simulink model "xpcserialbinarytest_orig"  (Simulink 7.1)
settings: Solver=FixedStepDiscrete  StartTime=0.0  StopTime=inf  RelTol=1e-3
InitFcn:
  | trun = .01;
libraries: xpclib x5, xpcutilitieslib x2, simulink x1
Description:
  | Serial Blocks Loopback Test Using Binary Encoding/Decoding
  | 
  | This model demonstrates the BINARY FIFO read block in a form that can be simulated without using any specific serial hardware.  The input to the FIFO write block is the concatenation of several pieces comprising two separate 'messages'.  The first message is the byte stream: [170, 1, N] and the second is [170 2 44 M] where N is an incrementing number and M is a decrementing number.  The initial '8' in the first constant is the number of elements that follow.  The '5' is an extraneous value that shows how the FIFO binary read will ignore extra information.
  | 
  | To run this test with real serial port hardware, replace the FIFO write block with the send/receive block with FIFO OUT that corresponds to your hardware from the xpclib rs232 section. Then feed the output signal back to the input with a wire to perform a loopback test.
settings Model: Creator=gweast  LastModifiedBy=Administrator  ExtModeArmWhenConnect=off  BufferReuse=off
settings DataIOCC: SaveOutput=off  SignalLogging=off  SaveTime=off
settings OptimizationCC: BlockReduction=off  OptimizeBlockIOStorage=off  BufferReuse=off  ExpressionFolding=off  FoldNonRolledExpr=off  LocalBlockOutputs=off
settings DebuggingCC: SaveWithParameterizedLinksMsg=none  SignalResolutionControl=TryResolveAllWithWarning  MultiTaskDSMMsg=warning  MultiTaskCondExecSysMsg=none  StrictBusMsg=None
settings HardwareCC: ProdIntDivRoundTo=Zero  ProdEndianess=LittleEndian  ProdHWDeviceType=Generic->32-bit x86 compatible
settings RTWCC: SystemTargetFile=xpctarget.tlc  TemplateMakefile=xpc_default_tmf  Description=xPC Target  ProcessScript=xpctarget_make_rtw_hook  IncludeERTFirstTime=on
settings xpcTargetCC: TargetFcnLib=ansi_tfl_tmw.mat  TargetFunctionLibrary=ANSI_C  CompOptLevelCompliant=off  PortableWordSizes=off  xPCisDownloadable=off

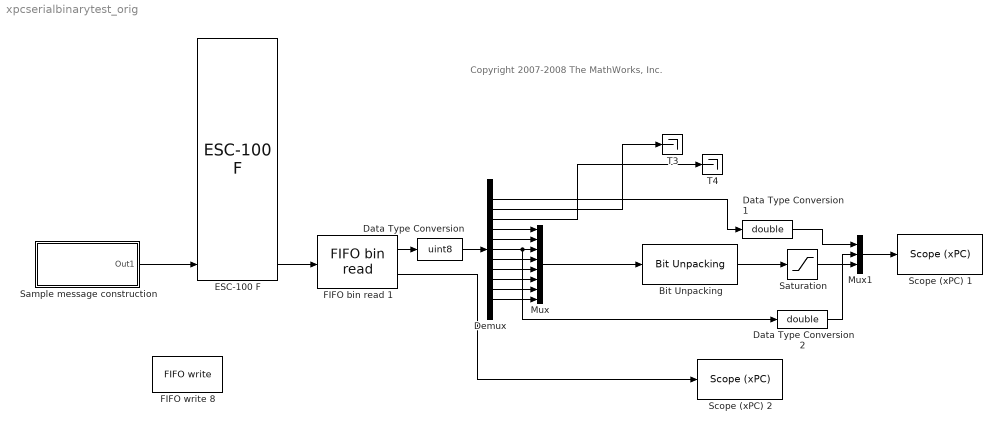
== system xpcserialbinarytest_orig ==
  note: Copyright 2007-2008 The MathWorks, Inc.
  "Bit Unpacking " : xpcutilitieslib/Bit Unpacking   SignExtend=off  MaskBitPatterns={[0:63]}  MaskPackDataType=uint8  MaskPackDataSize=[8]  MaskUnpackDataTypes={'double'}  MaskUnpackDataSizes={[1]}
  Data Type Conversion : DataTypeConversion  OutDataTypeMode=uint8  OutDataType=sfix(16)  OutScaling=2^0  OutDataTypeStr=uint8
  Data Type Conversion1 : DataTypeConversion  OutDataTypeMode=double  OutDataType=sfix(16)  OutScaling=2^0  OutDataTypeStr=double
  Data Type Conversion2 : DataTypeConversion  OutDataTypeMode=double  OutDataType=sfix(16)  OutScaling=2^0  OutDataTypeStr=double
  Demux : Demux  Outputs=11
  ESC-100 F : xpclib/RS232/Quatech/ESC-100/ESC-100 F  SystemSampleTime=-1  group=FIFO Setup  port=8  irqnum=10  slot=-1  baud1=9600  parity1=None  ndata1=8  nstop1=1  fifomode1=64 deep  rlevel1=half full  automode1=off  xmtfifosize1=1024  xmtdatatype1=8 bit uint null terminated  rcvfifosize1=1024  baud2=115200  parity2=None  ndata2=8  nstop2=1  fifomode2=64 deep  rlevel2=half full  automode2=on  xmtfifosize2=1024  xmtdatatype2=8 bit uint null terminated  rcvfifosize2=1024  baud3=115200  parity3=None  ndata3=8  nstop3=1  fifomode3=64 deep  rlevel3=half full  automode3=on  xmtfifosize3=1024  xmtdatatype3=8 bit uint null terminated  rcvfifosize3=1024  buad4=115200  parity4=None  ndata4=8  nstop4=1  fifomode4=64 deep  rlevel4=half full  automode4=on  xmtfifosize4=1024  xmtdatatype4=8 bit uint null terminated  rcvfifosize4=1024  baud5=115200  parity5=None  ndata5=8  nstop5=1  fifomode5=64 deep  rlevel5=half full  automode5=on  xmtfifosize5=1024  xmtdatatype5=8 bit uint null terminated  rcvfifosize5=1024  baud6=115200  parity6=None  ndata6=8  nstop6=1  fifomode6=64 deep  rlevel6=half full  automode6=on  xmtfifosize6=1024  xmtdatatype6=8 bit uint null terminated  rcvfifosize6=1024  baud7=115200  parity7=None  ndata7=8  nstop7=1  fifomode7=64 deep  rlevel7=half full  automode7=on  xmtfifosize7=1024  xmtdatatype7=8 bit uint null terminated  rcvfifosize7=1024  baud8=19200  parity8=None  ndata8=8  nstop8=1  fifomode8=64 deep  rlevel8=half full  automode8=on  xmtfifosize8=1024  xmtdatatype8=count+16 bit uint  rcvfifosize8=1024
  FIFO bin read 1 : xpclib/RS232/FIFO bin read   header={char([170, 1]), char([170,2])}  lengths=[10 4]  hold=Hold last output if no new data  enable=off  maxsize=10  outputtype=count+16 bit uint  sampletime=trun
  FIFO write 8 : xpclib/RS232/FIFO write   size=1024  inputtype=count+16 bit uint  present=off  sampletime=-1  id=XMT test
  Mux : Mux  Inputs=8
  Mux1 : Mux  Inputs=3
  Sample message construction : Subsystem
  Saturation : Saturate  UpperLimit=50  LowerLimit=-50  OutDataType=sfix(16)  OutScaling=2^0
  Scope (xPC) 1 : xpclib/Misc./Scope (xPC)   SystemSampleTime=-1  scopeno=2  scopetype=Target  autostart=on  viewmode=Graphical rolling  formatstr='%15.6f'  grid=on  ylimits=[0,0]  nosamples=512  noprepostsamples=0  interleave=1  triggermode=FreeRun  triggersignal=1  triggerlevel=0.0  triggerslope=Either  triggerscope=1  triggersample=0  filename=data.dat  mode=Lazy  writesize=512  autorestart=off
  Scope (xPC) 2 : xpclib/Misc./Scope (xPC)   SystemSampleTime=-1  scopeno=1  scopetype=Target  autostart=on  viewmode=Graphical rolling  formatstr='%15.6f'  grid=on  ylimits=[0,0]  nosamples=512  noprepostsamples=0  interleave=1  triggermode=FreeRun  triggersignal=1  triggerlevel=0.0  triggerslope=Either  triggerscope=1  triggersample=0  filename=data.dat  mode=Lazy  writesize=512  autorestart=off
  T3 : Terminator
  T4 : Terminator
  wires:
  FIFO bin read 1/2 -> Scope (xPC) 2/1
  Mux/1 -> "Bit Unpacking "/1
  Sample message construction/1(Out1) -> ESC-100 F/8
  ESC-100 F/8 -> FIFO bin read 1/1
  Mux1/1 -> Scope (xPC) 1/1
  "Bit Unpacking "/1 -> Saturation/1
  Data Type Conversion1/1 -> Mux1/1
  Saturation/1 -> Mux1/2
  Demux/4 -> Mux/1
  Demux/5 -> Mux/2
  Demux/6 -> Mux/3, Data Type Conversion2/1
  Demux/7 -> Mux/4
  FIFO bin read 1/1 -> Data Type Conversion/1
  Data Type Conversion/1 -> Demux/1
  Demux/8 -> Mux/5
  Demux/9 -> Mux/6
  Demux/10 -> Mux/7
  Demux/11 -> Mux/8
  Demux/3 -> T4/1
  Demux/2 -> T3/1
  Demux/1 -> Data Type Conversion1/1
  Data Type Conversion2/1 -> Mux1/3

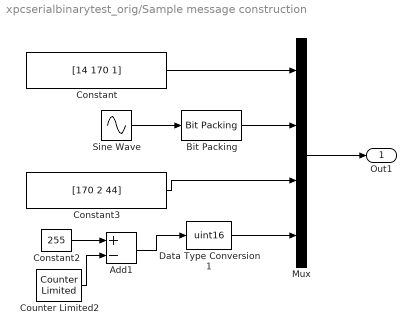
== system xpcserialbinarytest_orig/Sample message construction ==
  Add1 : Sum  Inputs=+-  OutDataType=sfix(16)  OutScaling=2^-10
  "Bit Packing " : xpcutilitieslib/Bit Packing   MaskBitPatterns={[0:63]}  MaskPackDataType=uint16  MaskPackDataSize=[8]
  Constant : Constant  Value=[14 170 1]  OutDataTypeMode=uint16  OutDataType=sfix(16)  OutScaling=2^0  OutDataTypeStr=uint16
  Constant2 : Constant  Value=255  OutDataType=sfix(16)  OutScaling=2^0
  Constant3 : Constant  Value=[170 2 44]  OutDataTypeMode=uint16  OutDataType=sfix(16)  OutScaling=2^0  OutDataTypeStr=uint16
  Counter Limited2 : simulink/Sources/Counter Limited  SystemSampleTime=-1  uplimit=255  tsamp=trun
  Data Type Conversion1 : DataTypeConversion  OutDataTypeMode=uint16  OutDataType=sfix(16)  OutScaling=2^0  OutDataTypeStr=uint16
  Mux : Mux
  Sine Wave : Sin  SampleTime=0
  Out1 : Outport  OutDataType=sfix(16)  OutScaling=2^0
  wires:
  Sine Wave/1 -> "Bit Packing "/1
  Constant/1 -> Mux/1
  Constant3/1 -> Mux/3
  "Bit Packing "/1 -> Mux/2
  Data Type Conversion1/1 -> Mux/4
  Mux/1 -> Out1/1
  Constant2/1 -> Add1/1
  Counter Limited2/1 -> Add1/2
  Add1/1 -> Data Type Conversion1/1
